simulink model "minmax_test"  (Simulink 7.2)
settings: Solver=FixedStepDiscrete  StartTime=0.0  StopTime=10.0  FixedStep=1.0  RelTol=1e-3
settings Model: Creator=arnaud  LastModifiedBy=arnaud
settings DataIOCC: SaveFormat=Structure

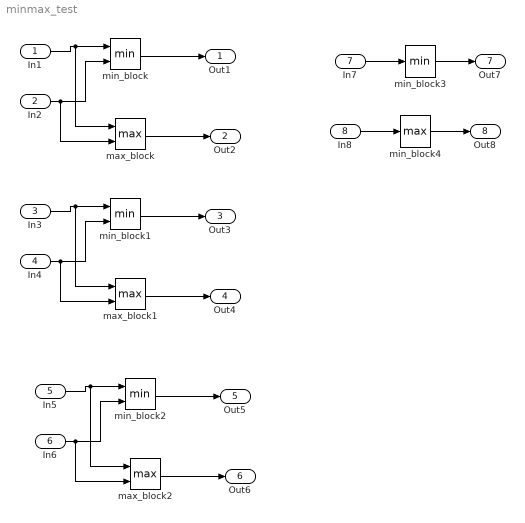
== system minmax_test ==
  In1 : Inport  OutDataType=sfix(16)  OutScaling=2^0
  In2 : Inport  Port=2  OutDataType=sfix(16)  OutScaling=2^0
  In3 : Inport  Port=3  PortDimensions=[2]  OutDataType=sfix(16)  OutScaling=2^0
  In4 : Inport  Port=4  PortDimensions=[2]  OutDataType=sfix(16)  OutScaling=2^0
  In5 : Inport  Port=5  PortDimensions=[2 2]  OutDataType=sfix(16)  OutScaling=2^0
  In6 : Inport  Port=6  PortDimensions=[2 2]  OutDataType=sfix(16)  OutScaling=2^0
  In7 : Inport  Port=7  PortDimensions=[3]  OutDataType=sfix(16)  OutScaling=2^0
  In8 : Inport  Port=8  PortDimensions=[7]  OutDataType=sfix(16)  OutScaling=2^0
  max_block : MinMax  Function=max  Inputs=2  OutDataType=sfix(16)  OutScaling=2^0
  max_block1 : MinMax  Function=max  Inputs=2  OutDataType=sfix(16)  OutScaling=2^0
  max_block2 : MinMax  Function=max  Inputs=2  OutDataType=sfix(16)  OutScaling=2^0
  min_block : MinMax  Inputs=2  OutDataType=sfix(16)  OutScaling=2^0
  min_block1 : MinMax  Inputs=2  OutDataType=sfix(16)  OutScaling=2^0
  min_block2 : MinMax  Inputs=2  OutDataType=sfix(16)  OutScaling=2^0
  min_block3 : MinMax  OutDataType=sfix(16)  OutScaling=2^0
  min_block4 : MinMax  Function=max  OutDataType=sfix(16)  OutScaling=2^0
  Out1 : Outport  OutDataType=sfix(16)  OutScaling=2^0
  Out2 : Outport  Port=2  OutDataType=sfix(16)  OutScaling=2^0
  Out3 : Outport  Port=3  OutDataType=sfix(16)  OutScaling=2^0
  Out4 : Outport  Port=4  OutDataType=sfix(16)  OutScaling=2^0
  Out5 : Outport  Port=5  OutDataType=sfix(16)  OutScaling=2^0
  Out6 : Outport  Port=6  OutDataType=sfix(16)  OutScaling=2^0
  Out7 : Outport  Port=7  OutDataType=sfix(16)  OutScaling=2^0
  Out8 : Outport  Port=8  OutDataType=sfix(16)  OutScaling=2^0
  wires:
  In1/1 -> min_block/1, max_block/1
  In2/1 -> min_block/2, max_block/2
  min_block/1 -> Out1/1
  max_block/1 -> Out2/1
  In3/1 -> min_block1/1, max_block1/1
  In4/1 -> min_block1/2, max_block1/2
  min_block1/1 -> Out3/1
  max_block1/1 -> Out4/1
  In5/1 -> min_block2/1, max_block2/1
  In6/1 -> min_block2/2, max_block2/2
  min_block2/1 -> Out5/1
  max_block2/1 -> Out6/1
  In7/1 -> min_block3/1
  min_block3/1 -> Out7/1
  In8/1 -> min_block4/1
  min_block4/1 -> Out8/1
